simulink subsystem "Vehicle_Driver"  (R2023b)
settings: Solver=VariableStepAuto  StartTime=0.0  StopTime=10.0  RelTol=1e-3
undefined symbols (not defined in the file or in its folder): DiscIntNeverNeededParam, driver, sim, track
libraries: slpidlib x2, simulink x1
settings Model: Creator=Inver  LastModifiedBy=Inver
settings OptimizationCC: ReuseModelBlockBuffer=off

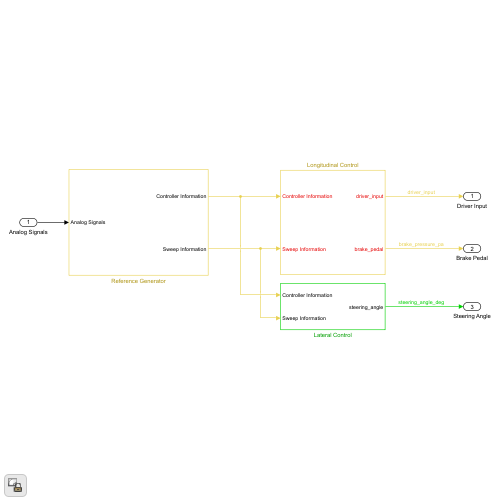
[thumbnail: Simulink's stored preview of the top-level diagram]
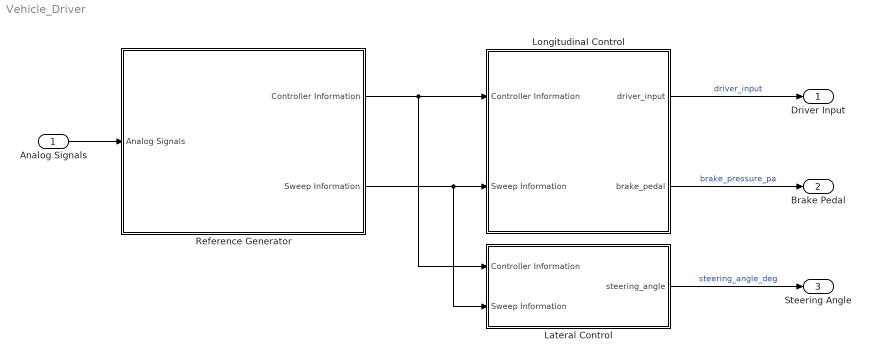
== system Vehicle_Driver ==
  Analog Signals : Inport
  Lateral Control : Subsystem
  Longitudinal Control : Subsystem
  Reference Generator : Subsystem
  Driver Input : Outport
  Brake Pedal : Outport  Port=2
  Steering Angle : Outport  Port=3
  wires:
  Analog Signals/1 -> Reference Generator/1(Analog Signals)
  Reference Generator/2(Sweep Information) -> Lateral Control/2(Sweep Information), Longitudinal Control/2(Sweep Information)
  Lateral Control/1(steering_angle) -> Steering Angle/1  "steering_angle_deg"
  Reference Generator/1(Controller Information) -> Lateral Control/1(Controller Information), Longitudinal Control/1(Controller Information)
  Longitudinal Control/2(brake_pedal) -> Brake Pedal/1  "brake_pressure_pa"
  Longitudinal Control/1(driver_input) -> Driver Input/1  "driver_input"

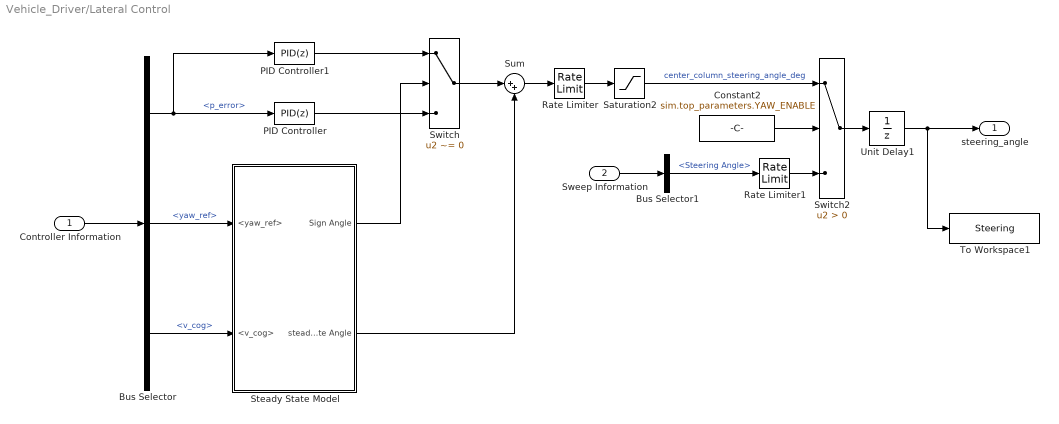
== system Vehicle_Driver/Lateral Control ==
  Controller Information : Inport
  Sweep Information : Inport  Port=2
  Bus Selector : BusSelector  OutputSignals=p_error,yaw_ref,v_cog
  Bus Selector1 : BusSelector  OutputSignals=Steering Angle
  Constant2 : Constant  Value=sim.top_parameters.YAW_ENABLE
  PID Controller : slpidlib/PID Controller  Controller=PID  Form=Parallel  TimeDomain=Discrete-time  UseExternalTs=off  SampleTime=-1  IntegratorMethod=Forward Euler  FilterMethod=Forward Euler  ControllerParametersSource=internal  P=driver.control.P_Straight_Adjust  I=0  UseKiTs=on  D=0  N=0  UseFilter=on  TunerSelectOption=Transfer Function Based (PID Tuner App)  InitialConditionSource=internal  InitialConditionForIntegrator=0  InitialConditionForFilter=0  DifferentiatorICPrevScaledInput=0  ExternalReset=none  TrackingMode=off  Kt=1  LimitOutput=on  SatLimitsSource=internal  UpperSaturationLimit=sim.range.MAX_STEERING_ADJUST*2  LowerSaturationLimit=-sim.range.MAX_STEERING_ADJUST*2  LinearizeAsGain=on  AntiWindupMode=none  Kb=1  LimitIntegrator=off  UpperIntegratorSaturationLimit=inf  LowerIntegratorSaturationLimit=-inf  POutMin=[]  POutMax=[]  IOutMin=[]  IOutMax=[]  DOutMin=[]  DOutMax=[]  NOutMin=[]  NOutMax=[]  SumOutMin=[]  SumOutMax=[]  SaturationOutMin=[]  SaturationOutMax=[]  PParamMin=[]  PParamMax=[]  IParamMin=[]  IParamMax=[]  DParamMin=[]  DParamMax=[]  NParamMin=[]  NParamMax=[]  KbParamMin=[]  KbParamMax=[]  KtParamMin=[]  KtParamMax=[]  KbOutMin=[]  KbOutMax=[]  KtOutMin=[]  KtOutMax=[]  IntegratorOutMin=[]  IntegratorOutMax=[]  FilterOutMin=[]  FilterOutMax=[]  SumI1OutMin=[]  SumI1OutMax=[]  SumI2OutMin=[]  SumI2OutMax=[]  SumI3OutMin=[]  SumI3OutMax=[]  SumI4OutMin=[]  SumI4OutMax=[]  SumDOutMin=[]  SumDOutMax=[]  DifferentiatorOutMin=[]  DifferentiatorOutMax=[]  FilterDiffOutCoefMin=[]  FilterDiffOutCoefMax=[]  ReciprocalOutMin=[]  ReciprocalOutMax=[]  SumDenOutMin=[]  SumDenOutMax=[]  SumNumOutMin=[]  SumNumOutMax=[]  DivideOutMin=[]  DivideOutMax=[]  UdiffTsProdOutMin=[]  UdiffTsProdOutMax=[]  NTsProdOutMin=[]  NTsProdOutMax=[]  UintegralTsProdOutMin=[]  UintegralTsProdOutMax=[]  UngainTsProdOutMin=[]  UngainTsProdOutMax=[]  ClampingZeroOutDataTypeStr=Inherit: Inherit via back propagation  ClampingZeroOutMin=[]  ClampingZeroOutMax=[]  FilterDenConstantOutDataTypeStr=Inherit: Inherit via back propagation  FilterDenConstantOutMin=[]  FilterDenConstantOutMax=[]  PCopyOutDataTypeStr=Inherit: Inherit via back propagation  PCopyOutMin=[]  PCopyOutMax=[]  NCopyOutDataTypeStr=Inherit: Inherit via back propagation  NCopyOutMin=[]  NCopyOutMax=[]  IntegratorContinuousStateAttributes=''  IntegratorStateMustResolveToSignalObject=off  IntegratorRTWStateStorageClass=Auto  FilterContinuousStateAttributes=''  FilterStateMustResolveToSignalObject=off  FilterRTWStateStorageClass=Auto  ParallelPVariant=InternalParameters  IdealPVariant=Disabled  IVariant=InternalParameters  DVariant=InternalParameters  IntegratorVariant=Discrete  SatVariant=Enabled  AWVariant=Passthrough  PCopyVariant=Disabled  TRVariant=Disabled  FdbkBlocksVariant=Forward  IdealPFdbkVariant=Disabled  SatFdbkVariant=Disabled  DerivativeFilterVariant=ForwardEulerFilter  NVariant=InternalParameters  NCopyVariant=Disabled  FilterICVariant=InternalICsFilter  IntegratorICVariant=InternalICs  ExternalResetVariant=Disabled  TRSumVariant=Passthrough  SumFdbkVariant=Disabled  SumVariant=Sum_PID  TsampFilterVariant=InternalTs  TsampNgainVariant=Passthrough  TsampIntegralVariant=Disabled_SignalSpec  ExternalSaturationOutDataTypeStr=Inherit: Same as second input
  PID Controller1 : slpidlib/PID Controller  Controller=PID  Form=Parallel  TimeDomain=Discrete-time  UseExternalTs=off  SampleTime=-1  IntegratorMethod=Forward Euler  FilterMethod=Forward Euler  ControllerParametersSource=internal  P=driver.control.P_Steering_Adjust  I=0  UseKiTs=on  D=0  N=0  UseFilter=on  TunerSelectOption=Transfer Function Based (PID Tuner App)  InitialConditionSource=internal  InitialConditionForIntegrator=0  InitialConditionForFilter=0  DifferentiatorICPrevScaledInput=0  ExternalReset=none  TrackingMode=off  Kt=1  LimitOutput=on  SatLimitsSource=internal  UpperSaturationLimit=sim.range.MAX_STEERING_ADJUST*2  LowerSaturationLimit=-sim.range.MAX_STEERING_ADJUST*2  LinearizeAsGain=on  AntiWindupMode=none  Kb=1  LimitIntegrator=off  UpperIntegratorSaturationLimit=inf  LowerIntegratorSaturationLimit=-inf  POutMin=[]  POutMax=[]  IOutMin=[]  IOutMax=[]  DOutMin=[]  DOutMax=[]  NOutMin=[]  NOutMax=[]  SumOutMin=[]  SumOutMax=[]  SaturationOutMin=[]  SaturationOutMax=[]  PParamMin=[]  PParamMax=[]  IParamMin=[]  IParamMax=[]  DParamMin=[]  DParamMax=[]  NParamMin=[]  NParamMax=[]  KbParamMin=[]  KbParamMax=[]  KtParamMin=[]  KtParamMax=[]  KbOutMin=[]  KbOutMax=[]  KtOutMin=[]  KtOutMax=[]  IntegratorOutMin=[]  IntegratorOutMax=[]  FilterOutMin=[]  FilterOutMax=[]  SumI1OutMin=[]  SumI1OutMax=[]  SumI2OutMin=[]  SumI2OutMax=[]  SumI3OutMin=[]  SumI3OutMax=[]  SumI4OutMin=[]  SumI4OutMax=[]  SumDOutMin=[]  SumDOutMax=[]  DifferentiatorOutMin=[]  DifferentiatorOutMax=[]  FilterDiffOutCoefMin=[]  FilterDiffOutCoefMax=[]  ReciprocalOutMin=[]  ReciprocalOutMax=[]  SumDenOutMin=[]  SumDenOutMax=[]  SumNumOutMin=[]  SumNumOutMax=[]  DivideOutMin=[]  DivideOutMax=[]  UdiffTsProdOutMin=[]  UdiffTsProdOutMax=[]  NTsProdOutMin=[]  NTsProdOutMax=[]  UintegralTsProdOutMin=[]  UintegralTsProdOutMax=[]  UngainTsProdOutMin=[]  UngainTsProdOutMax=[]  ClampingZeroOutDataTypeStr=Inherit: Inherit via back propagation  ClampingZeroOutMin=[]  ClampingZeroOutMax=[]  FilterDenConstantOutDataTypeStr=Inherit: Inherit via back propagation  FilterDenConstantOutMin=[]  FilterDenConstantOutMax=[]  PCopyOutDataTypeStr=Inherit: Inherit via back propagation  PCopyOutMin=[]  PCopyOutMax=[]  NCopyOutDataTypeStr=Inherit: Inherit via back propagation  NCopyOutMin=[]  NCopyOutMax=[]  IntegratorContinuousStateAttributes=''  IntegratorStateMustResolveToSignalObject=off  IntegratorRTWStateStorageClass=Auto  FilterContinuousStateAttributes=''  FilterStateMustResolveToSignalObject=off  FilterRTWStateStorageClass=Auto  ParallelPVariant=InternalParameters  IdealPVariant=Disabled  IVariant=InternalParameters  DVariant=InternalParameters  IntegratorVariant=Discrete  SatVariant=Enabled  AWVariant=Passthrough  PCopyVariant=Disabled  TRVariant=Disabled  FdbkBlocksVariant=Forward  IdealPFdbkVariant=Disabled  SatFdbkVariant=Disabled  DerivativeFilterVariant=ForwardEulerFilter  NVariant=InternalParameters  NCopyVariant=Disabled  FilterICVariant=InternalICsFilter  IntegratorICVariant=InternalICs  ExternalResetVariant=Disabled  TRSumVariant=Passthrough  SumFdbkVariant=Disabled  SumVariant=Sum_PID  TsampFilterVariant=InternalTs  TsampNgainVariant=Passthrough  TsampIntegralVariant=Disabled_SignalSpec  ExternalSaturationOutDataTypeStr=Inherit: Same as second input
  Rate Limiter : RateLimiter  RisingSlewLimit=sim.range.MAX_DTHETA_DRIVER  FallingSlewLimit=-sim.range.MAX_DTHETA_DRIVER  SampleTimeMode=inherited
  Rate Limiter1 : RateLimiter  RisingSlewLimit=sim.range.MAX_DTHETA_DRIVER  FallingSlewLimit=-sim.range.MAX_DTHETA_DRIVER  SampleTimeMode=inherited
  Saturation2 : Saturate  UpperLimit=sim.range.CENTER_STEER_ANGLE_MAX  LowerLimit=-sim.range.CENTER_STEER_ANGLE_MAX
  Steady State Model : Subsystem
  Sum : Sum  Inputs=|++
  Switch : Switch  Criteria=u2 ~= 0  SaturateOnIntegerOverflow=off  InputSameDT=off
  Switch2 : Switch  Criteria=u2 > Threshold  SaturateOnIntegerOverflow=off  InputSameDT=off
  To Workspace1 : ToWorkspace  VariableName=Steering  SaveFormat=Timeseries  SampleTime=-1
  Unit Delay1 : UnitDelay  SampleTime=sim.timing.duplicate  HasFrameUpgradeWarning=on
  steering_angle : Outport
  wires:
  Rate Limiter/1 -> Saturation2/1
  Controller Information/1 -> Bus Selector/1
  Bus Selector/1 -> PID Controller1/1, PID Controller/1  "<p_error>"
  PID Controller/1 -> Switch/3
  PID Controller1/1 -> Switch/1
  Switch/1 -> Sum/1
  Sum/1 -> Rate Limiter/1
  Saturation2/1 -> Switch2/1  "center_column_steering_angle_deg"
  Switch2/1 -> Unit Delay1/1
  Rate Limiter1/1 -> Switch2/3
  Constant2/1 -> Switch2/2
  Bus Selector1/1 -> Rate Limiter1/1  "<Steering Angle>"
  Sweep Information/1 -> Bus Selector1/1
  Unit Delay1/1 -> steering_angle/1, To Workspace1/1
  Steady State Model/1(Sign Angle) -> Switch/2
  Bus Selector/2 -> Steady State Model/1(<yaw_ref>)  "<yaw_ref>"
  Bus Selector/3 -> Steady State Model/2(<v_cog>)  "<v_cog>"
  Steady State Model/2(steady State Angle) -> Sum/2

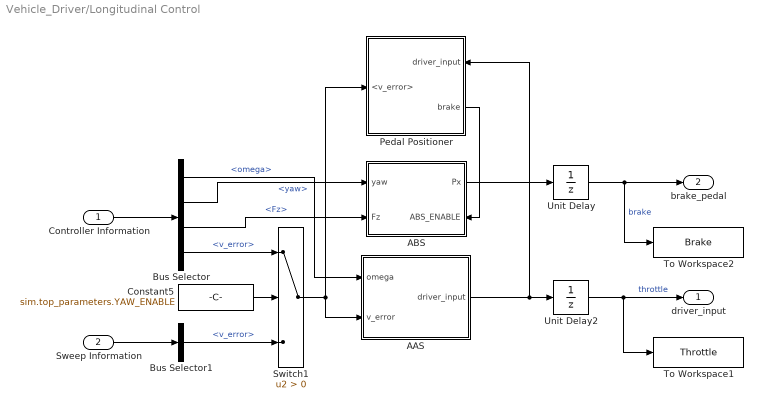
== system Vehicle_Driver/Longitudinal Control ==
  Controller Information : Inport
  Sweep Information : Inport  Port=2
  AAS : Subsystem
  ABS : Subsystem
      settings: PortSchema="{\"entries\":[{\"content\":{\"sides\":[{\"content\":{\"connectorIds\":[\"In1\",\"In2\"]},\"type\":\"ConnectorPlacement.EquallySpacedRectSide\",\"uuid\":\"05691032-3f39-4834-938a-125b9d9c5bbe\"},{\"content\":{\"connectorIds\":[\"Out1\",\"In3\"],\"side\":\"RIGHT\"},\"type\":\"ConnectorPlacement.EquallySpacedRectSide\",\"uuid\":\"b6342b01-7e0e-4c31-ae65-daa263149cd6\"},{\"content\":{\"connectorIds\":[],\"side\":\"TOP\"},\"type\":\"ConnectorPlacement.EquallySpacedRectSide\",\"uuid\":\"252d477f-1200-4151-9883-b9a128e2c38a\"}]},\"type\":\"ConnectorPlacement.EquallySpacedConnector\",\"uuid\":\"d67aaf26-3760-4411-918f-de910c7b3ed9\"}],\"packageUris\":[\"http://schema.mathworks.com/mf0/Connector/R2020b\"],\"version\":\"1.0\"}"
  Bus Selector : BusSelector  OutputSignals=omega,yaw,Fz,v_error
  Bus Selector1 : BusSelector  OutputSignals=v_error
  Constant5 : Constant  Value=sim.top_parameters.YAW_ENABLE
  Pedal Positioner : Subsystem
      settings: PortSchema="{\"entries\":[{\"content\":{\"sides\":[{\"content\":{\"connectorIds\":[\"In1\"]},\"type\":\"ConnectorPlacement.EquallySpacedRectSide\",\"uuid\":\"c84d1b45-47cb-44c3-9bb8-057964d890de\"},{\"content\":{\"connectorIds\":[\"In2\",\"Out1\"],\"side\":\"RIGHT\"},\"type\":\"ConnectorPlacement.EquallySpacedRectSide\",\"uuid\":\"136455d0-d36a-4818-af11-72b5a1b8c27c\"},{\"content\":{\"connectorIds\":[],\"side\":\"TOP\"},\"type\":\"ConnectorPlacement.EquallySpacedRectSide\",\"uuid\":\"42b2ce8c-2720-4fbc-908c-f7068b304798\"}]},\"type\":\"ConnectorPlacement.EquallySpacedConnector\",\"uuid\":\"ec27d525-5c9d-4748-8b13-bb528198656f\"}],\"packageUris\":[\"http://schema.mathworks.com/mf0/Connector/R2020b\"],\"version\":\"1.0\"}"
  Switch1 : Switch  Criteria=u2 > Threshold  SaturateOnIntegerOverflow=off  InputSameDT=off
  To Workspace1 : ToWorkspace  VariableName=Throttle  SaveFormat=Timeseries  SampleTime=-1
  To Workspace2 : ToWorkspace  VariableName=Brake  SaveFormat=Timeseries  SampleTime=-1
  Unit Delay : UnitDelay  InitialCondition=sim.IC.Brake_Pressure_IC  SampleTime=sim.timing.duplicate  HasFrameUpgradeWarning=on
  Unit Delay2 : UnitDelay  InitialCondition=sim.IC.driver_input_IC  SampleTime=sim.timing.duplicate  HasFrameUpgradeWarning=on
  driver_input : Outport  PortDimensions=1
  brake_pedal : Outport  Port=2
  wires:
  Controller Information/1 -> Bus Selector/1
  Constant5/1 -> Switch1/2
  Sweep Information/1 -> Bus Selector1/1
  Bus Selector1/1 -> Switch1/3  "<v_error>"
  Bus Selector/4 -> Switch1/1  "<v_error>"
  Switch1/1 -> Pedal Positioner/1(<v_error>), AAS/2(v_error)
  AAS/1(driver_input) -> Pedal Positioner/2(driver_input), Unit Delay2/1
  ABS/1(Px) -> Unit Delay/1
  Pedal Positioner/1(brake) -> ABS/3(ABS_ENABLE)
  Bus Selector/3 -> ABS/2(Fz)  "<Fz>"
  Unit Delay2/1 -> To Workspace1/1, driver_input/1  "throttle"
  Unit Delay/1 -> To Workspace2/1, brake_pedal/1  "brake"
  Bus Selector/2 -> ABS/1(yaw)  "<yaw>"
  Bus Selector/1 -> AAS/1(omega)  "<omega>"

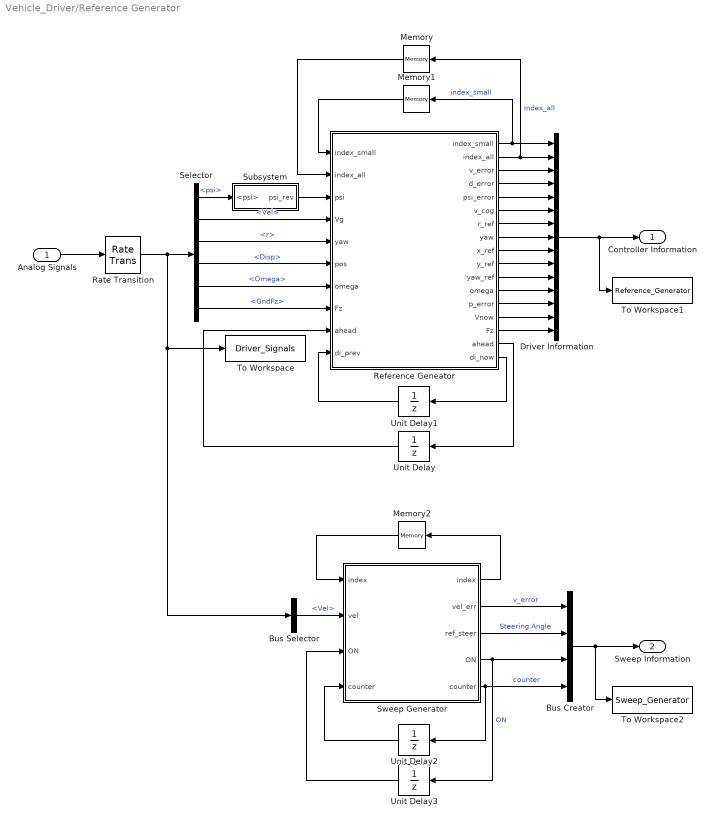
== system Vehicle_Driver/Reference Generator ==
  Analog Signals : Inport
  Bus Creator : BusCreator  Inputs=4
  Bus Selector : BusSelector  OutputSignals=Vel
  Driver Information : BusCreator  Inputs=15
  Memory : Memory  InitialCondition=1
  Memory1 : Memory  InitialCondition=1
  Memory2 : Memory  InitialCondition=1
  Rate Transition : RateTransition  OutPortSampleTime=sim.timing.duplicate
  Reference Geneator : MATLAB Function  TreatAsAtomicUnit=on  SystemSampleTime=sim.timing.duplicate
  Selector : BusSelector  OutputSignals=psi,Vel,r,Disp,Omega,GndFz
  Subsystem : Subsystem
  Sweep Generator : MATLAB Function  TreatAsAtomicUnit=on  SystemSampleTime=sim.timing.duplicate
  To Workspace : ToWorkspace  VariableName=Driver_Signals  SaveFormat=Timeseries  SampleTime=-1
  To Workspace1 : ToWorkspace  VariableName=Reference_Generator  SaveFormat=Timeseries  SampleTime=-1
  To Workspace2 : ToWorkspace  VariableName=Sweep_Generator  SaveFormat=Timeseries  SampleTime=-1
  Unit Delay : UnitDelay  SampleTime=-1  HasFrameUpgradeWarning=on
  Unit Delay1 : UnitDelay  InitialCondition=1000  SampleTime=-1  HasFrameUpgradeWarning=on
  Unit Delay2 : UnitDelay  SampleTime=-1  HasFrameUpgradeWarning=on
  Unit Delay3 : UnitDelay  InitialCondition=1  SampleTime=-1  HasFrameUpgradeWarning=on
  Controller Information : Outport
  Sweep Information : Outport  Port=2
  wires:
  Analog Signals/1 -> Rate Transition/1
  Selector/1 -> Subsystem/1(<psi>)  "<psi>"
  Reference Geneator/4(d_error) -> Driver Information/4
  Driver Information/1 -> Controller Information/1, To Workspace1/1
  Selector/2 -> Reference Geneator/4(Vg)  "<Vel>"
  Reference Geneator/3(v_error) -> Driver Information/3
  Reference Geneator/6(v_cog) -> Driver Information/6
  Subsystem/1(psi_rev) -> Reference Geneator/3(psi)
  Reference Geneator/5(psi_error) -> Driver Information/5
  Reference Geneator/2(index_all) -> Driver Information/2, Memory/1  "index_all"
  Memory/1 -> Reference Geneator/2("index_all ")
  Reference Geneator/7(r_ref) -> Driver Information/7
  Reference Geneator/8(yaw) -> Driver Information/8
  Reference Geneator/16(ahead) -> Unit Delay/1
  Unit Delay/1 -> Reference Geneator/9("ahead ")
  Reference Geneator/12(omega) -> Driver Information/12
  Reference Geneator/9(x_ref) -> Driver Information/9
  Reference Geneator/10(y_ref) -> Driver Information/10
  Selector/3 -> Reference Geneator/5("yaw ")  "<r>"
  Selector/4 -> Reference Geneator/6(pos)  "<Disp>"
  Reference Geneator/11(yaw_ref) -> Driver Information/11
  Memory1/1 -> Reference Geneator/1("index_small ")
  Reference Geneator/17(di_now) -> Unit Delay1/1
  Unit Delay1/1 -> Reference Geneator/10(di_prev)
  Selector/5 -> Reference Geneator/7("omega ")  "<Omega>"
  Reference Geneator/13(p_error) -> Driver Information/13
  Reference Geneator/14(Vnow) -> Driver Information/14
  Reference Geneator/1(index_small) -> Memory1/1, Driver Information/1  "index_small"
  Sweep Generator/4(ON) -> Bus Creator/3, Unit Delay3/1  "ON"
  Sweep Generator/5(counter) -> Bus Creator/4, Unit Delay2/1  "counter"
  Unit Delay3/1 -> Sweep Generator/3("ON ")
  Memory2/1 -> Sweep Generator/1("index ")
  Unit Delay2/1 -> Sweep Generator/4("counter ")
  Bus Creator/1 -> To Workspace2/1, Sweep Information/1
  Sweep Generator/3(ref_steer) -> Bus Creator/2  "Steering Angle"
  Bus Selector/1 -> Sweep Generator/2(vel)  "<Vel>"
  Sweep Generator/2(vel_err) -> Bus Creator/1  "v_error"
  Sweep Generator/1(index) -> Memory2/1
  Selector/6 -> Reference Geneator/8("Fz ")  "<GndFz>"
  Reference Geneator/15(Fz) -> Driver Information/15
  Rate Transition/1 -> Bus Selector/1, To Workspace/1, Selector/1

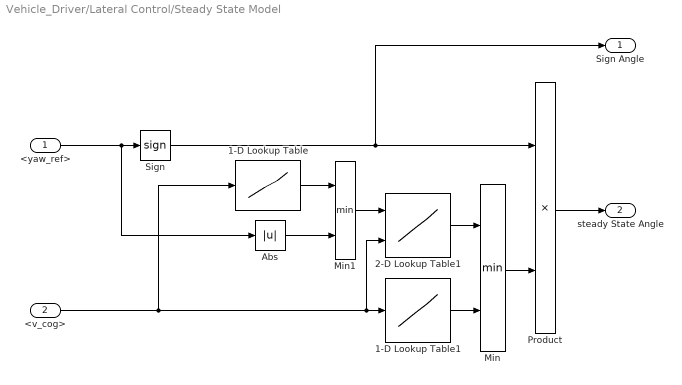
== system Vehicle_Driver/Lateral Control/Steady State Model ==
  <yaw_ref> : Inport
  <v_cog> : Inport  Port=2
  1-D Lookup Table : Lookup_n-D  NumberOfTableDimensions=1  BreakpointsForDimension1=driver.control.max_v_bp  Table=driver.control.max_yaw_table  ExtrapMethod=Clip  InternalRulePriority=Speed  RndMeth=Simplest
  1-D Lookup Table1 : Lookup_n-D  NumberOfTableDimensions=1  BreakpointsForDimension1=driver.control.max_v_bp  Table=driver.control.max_theta_table  InternalRulePriority=Speed  RndMeth=Simplest
  2-D Lookup Table1 : Lookup_n-D  BreakpointsForDimension1=driver.control.max_y_bp  BreakpointsForDimension2=driver.control.max_v_bp  Table=driver.control.steering_angle_table  ExtrapMethod=Clip  InternalRulePriority=Speed  RndMeth=Simplest
      settings: InputPortMap=u0,u1
  Abs : Abs  SaturateOnIntegerOverflow=off
  Min : MinMax  Inputs=2
  Min1 : MinMax  Inputs=2
  Product : Product
  Sign : Signum
  Sign Angle : Outport
  steady State Angle : Outport  Port=2
  wires:
  Sign/1 -> Sign Angle/1, Product/1
  1-D Lookup Table1/1 -> Min/2
  Min1/1 -> 2-D Lookup Table1/1
  <yaw_ref>/1 -> Abs/1, Sign/1
  <v_cog>/1 -> 2-D Lookup Table1/2, 1-D Lookup Table1/1, 1-D Lookup Table/1
  Min/1 -> Product/2
  Abs/1 -> Min1/2
  2-D Lookup Table1/1 -> Min/1
  Product/1 -> steady State Angle/1
  1-D Lookup Table/1 -> Min1/1

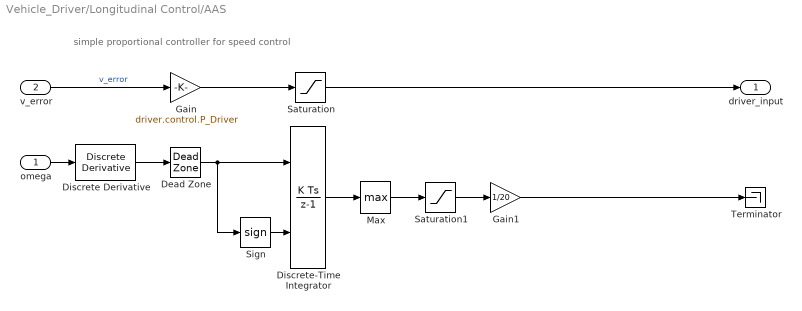
== system Vehicle_Driver/Longitudinal Control/AAS ==
  note: simple proportional controller for speed control
  omega : Inport
  v_error : Inport  Port=2
  Dead Zone : DeadZone  LowerValue=-15  UpperValue=15
  Discrete Derivative : simulink/Discrete/Discrete Derivative  gainval=1.0  ICPrevScaledInput=0.0  OutMin=[]  OutMax=[]  OutDataType=fixdt(1, 16)  OutScaling=2^-10  DoSatur=off
  Discrete-Time Integrator : DiscreteIntegrator  ExternalReset=either  SampleTime=-1  ICPrevOutput=DiscIntNeverNeededParam  ICPrevScaledInput=DiscIntNeverNeededParam
  Gain : Gain  Gain=driver.control.P_Driver
  Gain1 : Gain  Gain=1/20
  Max : MinMax  Function=max
  Saturation : Saturate  UpperLimit=sim.range.Max_Driver_Input  LowerLimit=sim.range.Min_Driver_Input
  Saturation1 : Saturate  UpperLimit=inf  LowerLimit=0
  Sign : Signum
  Terminator : Terminator
  driver_input : Outport
  wires:
  Gain/1 -> Saturation/1
  v_error/1 -> Gain/1  "v_error"
  omega/1 -> Discrete Derivative/1
  Discrete Derivative/1 -> Dead Zone/1
  Discrete-Time Integrator/1 -> Max/1
  Dead Zone/1 -> Sign/1, Discrete-Time Integrator/1
  Sign/1 -> Discrete-Time Integrator/2
  Max/1 -> Saturation1/1
  Saturation1/1 -> Gain1/1
  Gain1/1 -> Terminator/1
  Saturation/1 -> driver_input/1

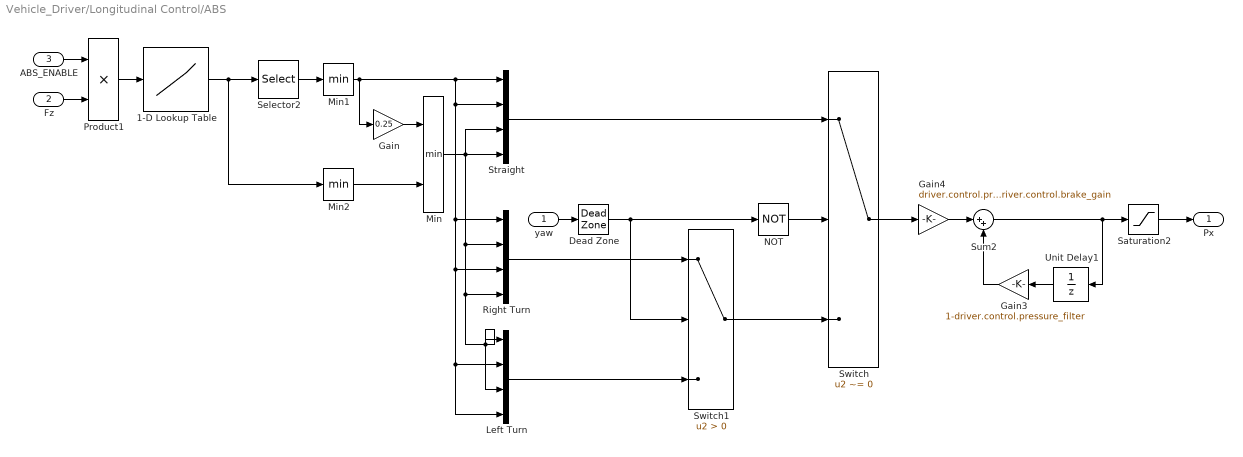
== system Vehicle_Driver/Longitudinal Control/ABS ==
  yaw : Inport
  Fz : Inport  Port=2
  ABS_ENABLE : Inport  Port=3
  1-D Lookup Table : Lookup_n-D  NumberOfTableDimensions=1  BreakpointsForDimension1=[0;200;400;600;800;1000;1200]  Table=[0;0;500000;750000;1000000;2000000;2000000]  ExtrapMethod=Clip  InternalRulePriority=Speed  RndMeth=Simplest
  Dead Zone : DeadZone  LowerValue=-0.1  UpperValue=0.1
  Gain : Gain  Gain=0.25
  Gain3 : Gain  Gain=1-driver.control.pressure_filter
  Gain4 : Gain  Gain=driver.control.pressure_filter*sim.top_parameters.YAW_ENABLE*driver.control.brake_gain
  Left Turn : Mux
  Min : MinMax  Inputs=2
  Min1 : MinMax
  Min2 : MinMax
  NOT : Logic  Operator=NOT  IconShape=distinctive  AllPortsSameDT=off  OutDataTypeStr=boolean
  Product1 : Product
  Right Turn : Mux
  Saturation2 : Saturate  UpperLimit=sim.range.Max_Brake_Pressure  LowerLimit=sim.range.Min_Brake_Pressure
  Selector2 : Selector  InputPortWidth=4  IndexOptions=Index vector (dialog)  Indices=[1 2]  OutputSizes=1
  Straight : Mux
  Sum2 : Sum  Inputs=|++
  Switch : Switch  Criteria=u2 ~= 0  SaturateOnIntegerOverflow=off  InputSameDT=off
  Switch1 : Switch  Criteria=u2 > Threshold  SaturateOnIntegerOverflow=off  InputSameDT=off
  Unit Delay1 : UnitDelay  SampleTime=-1  HasFrameUpgradeWarning=on
  Px : Outport
  wires:
  ABS_ENABLE/1 -> Product1/1
  Gain3/1 -> Sum2/2
  Unit Delay1/1 -> Gain3/1
  Gain4/1 -> Sum2/1
  Sum2/1 -> Saturation2/1, Unit Delay1/1
  Fz/1 -> Product1/2
  Saturation2/1 -> Px/1
  Product1/1 -> 1-D Lookup Table/1
  Gain/1 -> Min/1
  1-D Lookup Table/1 -> Min2/1, Selector2/1
  Selector2/1 -> Min1/1
  Min1/1 -> Straight/2, Right Turn/3, Left Turn/2, Left Turn/4, Right Turn/1, Straight/1, Gain/1
  Min/1 -> Left Turn/1, Left Turn/3, Right Turn/4, Right Turn/2, Straight/4, Straight/3
  Min2/1 -> Min/2
  Straight/1 -> Switch/1
  Left Turn/1 -> Switch1/3
  Right Turn/1 -> Switch1/1
  Switch1/1 -> Switch/3
  Switch/1 -> Gain4/1
  yaw/1 -> Dead Zone/1
  Dead Zone/1 -> Switch1/2, NOT/1
  NOT/1 -> Switch/2

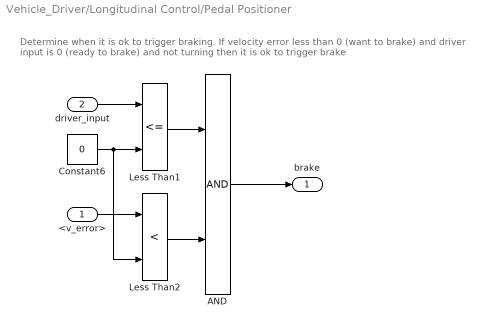
== system Vehicle_Driver/Longitudinal Control/Pedal Positioner ==
  note: Determine when it is ok to trigger braking. If velocity error less than 0 (want to brake) and driver input is 0 (ready to brake) and not turning then it is ok to trigger brake
  <v_error> : Inport
  driver_input : Inport  Port=2
  AND : Logic  IconShape=distinctive  AllPortsSameDT=off  OutDataTypeStr=boolean
  Constant6 : Constant  Value=0
  Less Than1 : RelationalOperator  Operator=<=  OutDataTypeStr=boolean  RndMeth=Simplest  InputSameDT=off
  Less Than2 : RelationalOperator  Operator=<  OutDataTypeStr=boolean  RndMeth=Simplest  InputSameDT=off
  brake : Outport
  wires:
  Constant6/1 -> Less Than1/2, Less Than2/2
  AND/1 -> brake/1
  Less Than2/1 -> AND/2
  <v_error>/1 -> Less Than2/1
  Less Than1/1 -> AND/1
  driver_input/1 -> Less Than1/1

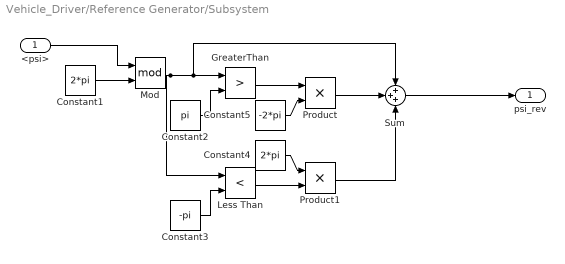
== system Vehicle_Driver/Reference Generator/Subsystem ==
  <psi> : Inport
  Constant1 : Constant  Value=2*pi
  Constant2 : Constant  Value=pi
  Constant3 : Constant  Value=-pi
  Constant4 : Constant  Value=2*pi
  Constant5 : Constant  Value=-2*pi
  GreaterThan : RelationalOperator  Operator=>  OutDataTypeStr=boolean  RndMeth=Simplest  InputSameDT=off
  Less Than : RelationalOperator  Operator=<  OutDataTypeStr=boolean  RndMeth=Simplest  InputSameDT=off
  Mod : Math  Operator=mod
  Product : Product
  Product1 : Product
  Sum : Sum  Inputs=+++
  psi_rev : Outport
  wires:
  Product1/1 -> Sum/3
  Less Than/1 -> Product1/2
  GreaterThan/1 -> Product/1
  Mod/1 -> GreaterThan/1, Sum/1, Less Than/1
  Constant1/1 -> Mod/2
  Constant5/1 -> Product/2
  Constant3/1 -> Less Than/2
  Constant4/1 -> Product1/1
  Constant2/1 -> GreaterThan/2
  Product/1 -> Sum/2
  Sum/1 -> psi_rev/1
  <psi>/1 -> Mod/1

== matlab function Vehicle_Driver/Reference Generator/Reference Geneator ==
  data: index_small output size=1; index_all output; index_small input size=1; index_all input size=1; psi input; Vg input; yaw input; pos input; omega input; Fz input; v_error output; d_error output; psi_error output; v_cog output; r_ref output; yaw output; x_ref output; y_ref output; yaw_ref output; omega output; p_error output; Vnow output; Fz output; ahead output; ahead input; driver parameter; di_prev input; sim parameter; di_now output; track parameter
function [index_small,index_all, v_error, d_error, psi_error, v_cog, r_ref, yaw, x_ref, y_ref, yaw_ref, omega, p_error,Vnow, Fz, ahead, di_now] = ref_gen(index_small,index_all, psi, Vg, yaw, pos, omega, Fz, ahead, driver, di_prev, sim, track)
%% Extract Data
num_elem = length(track.selected_track(:,2));

if index_all+driver.vision.dIndex <= num_elem
    Y_all = track.selected_track(index_all:index_all+driver.vision.dIndex,2);
    X_all = track.selected_track(index_all:index_all+driver.vision.dIndex,3);
else
    Y_all = track.selected_track(index_all:index_all+driver.vision.dIndex,2);
    X_all = track.selected_track(index_all:index_all+driver.vision.dIndex,3);
%     Y_all = pos(2);
%     X_all = pos(1);
end

Vmax_now = track.selected_maxvm(index_small,3);
num_elem = length(track.selected_maxvm(:,1));

if num_elem > index_small
    Vmax_next = track.selected_maxvm(index_small+1,3);
    d_next = track.selected_maxvm(index_small+1,1);
else
    Vmax_next = Vmax_now;
    d_next = 100;
end

%% Determine Reference Point
d_error_all = sqrt((Y_all - pos(2)).^2 + (X_all - pos(1)).^2);
[min_d, min_index] = min(d_error_all);
index_all = index_all + min_index - 1;

%% Aquire Reference Values
y_ref = track.selected_track(index_all, 2);
x_ref = track.selected_track(index_all, 3);
y_ref_next = track.selected_track(index_all+5, 2);
x_ref_next = track.selected_track(index_all+5, 3);
r_ref = track.selected_track(index_all, 4);
turn_ref = track.selected_track(index_all, 5);
psi_ref = track.selected_track(index_all, 8);
di_now = track.selected_track(index_all, 9);

%% Velocity Error
v_cog = sqrt((Vg(1)^2) + (Vg(2)^2));

if ahead
    di = (di_now*driver.vision.dx) + d_next;
else
    di = di_now*driver.vision.dx;
end

det = v_cog^2 + (2*driver.control.axb*di);

if det < 0
    Vnext = 0;
else
    Vnext = sqrt(det);
end

% straight driving simulation
% d_now = pos(1);
% d_later = selected_maxvm(index_small,4);
% dS = d_now - d_later;
% det = v_cog^2 - (2*axb*dS);
% 
% if det > 0
%     Vnext = sqrt(det);
% else
%     Vnext = 0;
% end

increment = 0;

% if (abs(Vmax_next - Vnext) < 0.1) && (Vmax_now > Vmax_next) && (~ahead)
%     Vnow = Vmax_next;
%     index_small = index_small + 1;
%     ahead = 1;
%     increment = 1;
if ((di_now - di_prev) > 0) && ~ahead
    Vnow = Vmax_next;
    index_small = index_small + 1;
else
    Vnow = Vmax_now;
end

if ((di_now - di_prev) > 0) && ~increment
    ahead = 0;
end

if (Vnext + 0.5 < Vnow) && (track.selected_maxvm(index_small,1) ~= 40)
    Vnow = 50;
end

if Vnow > 14
    v_error = Vnow - v_cog; % - 2
else
    v_error = Vnow - v_cog; % - 1
end

%% Turning Radius Error
r_IC = abs(v_cog / yaw);
r_error = turn_ref *  ((1 / r_ref) - (1 / r_IC));

if r_ref == inf
    yaw_ref = 0;
else
    yaw_ref = turn_ref * v_cog / r_ref;
end

%% Angle Error
sign_steer = 1;

if (abs(psi - psi_ref) > pi) && (sign(psi) ~= sign(psi_ref))
    if psi < 0
        sign_steer = -1;
    end
elseif (psi > psi_ref)
    sign_steer = -1;   
end

if abs(psi_ref - psi) < pi
    psi_error = sign_steer * abs(psi_ref - psi) / sim.constant.deg2rad;
else
    psi_error = sign_steer * ((pi - abs(psi_ref)) + (pi - abs(psi))) / sim.constant.deg2rad;
end

%% Distance Error
% Determine Vehicle Quadrant
if (pos(2) - y_ref) > driver.vision.q_thresh
   if (pos(1) - x_ref) > driver.vision.q_thresh
       Qc = 5;
   elseif (pos(1) - x_ref) < -driver.vision.q_thresh
       Qc = 11;
   else
       Qc = 4;
   end
elseif (pos(2) - y_ref) < -driver.vision.q_thresh
   if (pos(1) - x_ref) > driver.vision.q_thresh
       Qc = 7;
   elseif (pos(1) - x_ref) < -driver.vision.q_thresh
       Qc = 9;
   else
       Qc = 8;
   end
else
   if (pos(1) - x_ref) > driver.vision.q_thresh
       Qc = 6;
   elseif (pos(1) - x_ref) < -driver.vision.q_thresh
       Qc = 10;
   else
       Qc = 0;
   end
end

% Determine Next Reference Point Quadrant
if y_ref_next > y_ref
   if x_ref_next > x_ref
       Qn = 5;
   elseif x_ref_next < x_ref
       Qn = 11;
   else
       Qn = 4;
   end
elseif y_ref_next < y_ref
   if x_ref_next > x_ref
       Qn = 7;
   elseif x_ref_next < x_ref
       Qn = 9;
   else
       Qn = 8;
   end
else
   if x_ref_next > x_ref
       Qn = 6;
   elseif x_ref_next < x_ref
       Qn = 10;
   else
       Qn = 0;
   end
end

% Determine Sign for Distance Error
if Qc == 0
   sign_distance = 0;
elseif (abs(x_ref_next - x_ref) == abs(pos(1) - x_ref)) && (abs(y_ref_next - y_ref) == abs(pos(2) - y_ref))
   sign_distance = 0;
elseif ((Qc ~= Qn) && (driver.vision.indicies(Qc+4) ~= Qn))
    if (driver.vision.indicies(Qc+1) == driver.vision.indicies(Qn)) || (driver.vision.indicies(Qc+2) == driver.vision.indicies(Qn)) || (driver.vision.indicies(Qc+3) == driver.vision.indicies(Qn))
        sign_distance = -1;
    else
        sign_distance = 1;
    end
else
    if driver.vision.indicies(Qc) == 1 || driver.vision.indicies(Qc) == 3
        y_axis = y_ref;
    elseif driver.vision.indicies(Qc) == 4
        y_axis = y_ref + 1;
    else
        y_axis = y_ref - 1;
    end
    
    if driver.vision.indicies(Qc) == 2 || driver.vision.indicies(Qc) == 4
        x_axis = x_ref;
    elseif driver.vision.indicies(Qc) == 1
        x_axis = x_ref + 1;
    else
        x_axis = x_ref - 1;
    end
    
    axis_coordiantes = [y_axis, x_axis];
    ref_coordiantes = [y_ref, x_ref];
    next_ref_coordinates = [y_ref_next, x_ref_next];
    vehicle_coordinates = [pos(2), pos(1)];
    
    ref_vec = axis_coordiantes - ref_coordiantes;
    veh_vec = vehicle_coordinates - ref_coordiantes;
    next_ref = next_ref_coordinates - ref_coordiantes;
    
    theta_veh_ref = acos(dot(ref_vec, veh_vec) / (norm(ref_vec)*norm(veh_vec)));
    theta_next_ref = acos(dot(ref_vec, next_ref) / (norm(ref_vec)*norm(next_ref)));
    
    if theta_veh_ref < theta_next_ref
        sign_distance = 1;
    else
        sign_distance = -1;
    end
end

d_error = sign_distance * min_d;

%% Combined Purtubation Error
if (sign_distance~=sign(psi_error)) && (d_error~=0)
    p_error = d_error;
else
    p_error = psi_error;
end

end

== matlab function Vehicle_Driver/Reference Generator/Sweep Generator ==
  data: index input; index output; vel input; ON input; sim parameter; driver parameter; counter input; vel_err output; ref_steer output; ON output; counter output; track parameter
function [index, vel_err,ref_steer, ON, counter] = fcn(index, vel, ON, sim, driver, counter, track)

% Update Control Output
ref_vel = track.selected_sweep(index, 1);
ref_steer = track.selected_sweep(index, 2);
vel_err = ref_vel - norm([vel(1) vel(2)]);
counter = counter + 1;

% Update Scenario
if ((counter*sim.timing.duplicate) == driver.control.dt_ON && ON) || ((counter*sim.timing.duplicate) == driver.control.dt_OFF && ~ON)
    index = index + 1;
    counter = 0;

    if (track.selected_sweep(index, 2) == 0 && index > 1)
        ON = double(~ON);
    end

end
